simulink model "DoubleAdaptiveCBF3D"  (R2019a)
settings: Solver=ode4  StartTime=0.0  StopTime=80  FixedStep=0.001  RelTol=1e-3
values from neighbouring files (symbols this model uses):
  ddK_est0 = zeros(n,1)    [init6CBF3D.m]
  ddpref_est0 = zeros(3*n,1)    [init6CBF3D.m]
  dK0 = zeros(n,1)    [init6CBF3D.m]
  dK_est0 = zeros(n,1)    [init6CBF3D.m]
  dp0 = zeros(3*n,1)    [init6CBF3D.m]
  dpref0 = zeros(3*n,1)    [init6CBF3D.m]
  dpref_est0 = zeros(3*n,1)    [init6CBF3D.m]
  K0 = ones(n,1)    [init6CBF3D.m]
  K_est0 = ones(n,1)    [init6CBF3D.m]
  K_min = 0.3    [init6CBF3D.m]
  K_ref = 1    [init6CBF3D.m]
  obss = [ 15  16 -5  19   0  8  4 ... (first row only)    [init6CBF3D.m]
  p0 = rand(3*n,1)    [init6CBF3D.m]
  pd = reshape(pd',3*n,1)    [init6CBF3D.m]
  pref0 = zeros(3*n,1)    [init6CBF3D.m]
  pref_est0 = zeros(3*n,1)    [init6CBF3D.m]
  topology = sign(abs(LL))    [init6CBF3D.m]
libraries: commchan3 x1, cstblocks x1
settings Model: Creator=zxz  LastModifiedBy=zxz

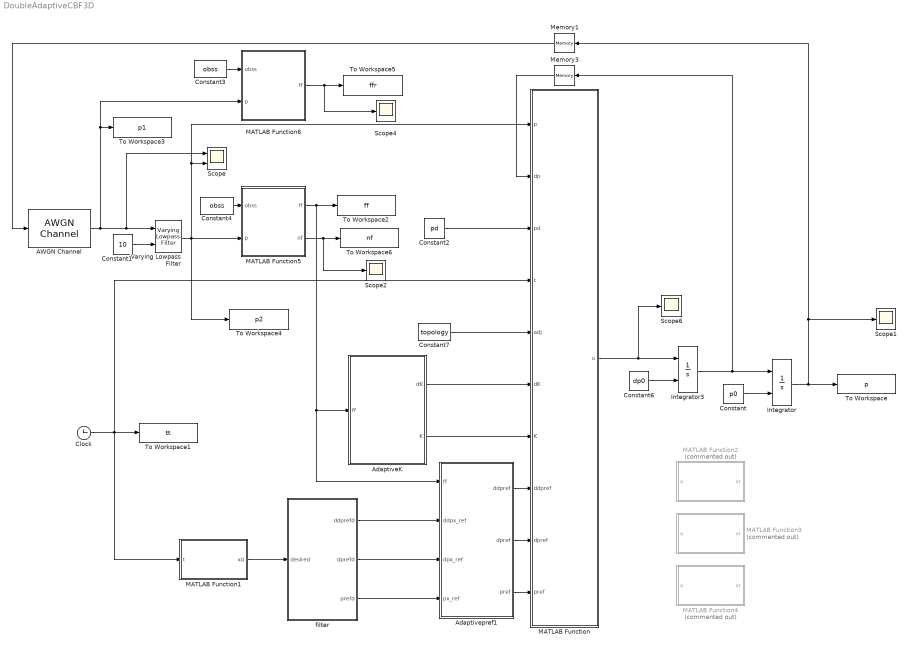
== system DoubleAdaptiveCBF3D ==
  AWGN Channel : commchan3/AWGN Channel  InputProcessing=Columns as channels (frame based)  seed=67  noiseMode="Signal to noise ratio  (Eb/No)"  EbNodB=65  EsNodB=10  SNRdB=10  bitsPerSym=1  Ps=1  Tsym=1  variance=1
      settings: SourceProductName=Communications Toolbox
  AdaptiveK : Subsystem
  Adaptivepref1 : Subsystem
  Clock : Clock
  Constant : Constant  Value=p0
  Constant1 : Constant  Value=10
  Constant2 : Constant  Value=pd
  Constant3 : Constant  Value=obss
  Constant4 : Constant  Value=obss
  Constant6 : Constant  Value=dp0
  Constant7 : Constant  Value=topology
  Integrator : Integrator  InitialConditionSource=external
  Integrator3 : Integrator  InitialConditionSource=external
  MATLAB Function : MATLAB Function  TreatAsAtomicUnit=on
  MATLAB Function1 : MATLAB Function  TreatAsAtomicUnit=on
  MATLAB Function2 : MATLAB Function  Commented=on  TreatAsAtomicUnit=on
  MATLAB Function3 : MATLAB Function  Commented=on  TreatAsAtomicUnit=on
  MATLAB Function4 : MATLAB Function  Commented=on  TreatAsAtomicUnit=on
  MATLAB Function5 : MATLAB Function  TreatAsAtomicUnit=on
  MATLAB Function6 : MATLAB Function  TreatAsAtomicUnit=on
  Memory1 : Memory
  Memory3 : Memory
  Scope : Scope  NumInputPorts=2
  Scope{1..2,4,6} (4 alike) : Scope
  To Workspace : ToWorkspace  VariableName=p  SampleTime=-1
  To Workspace1 : ToWorkspace  VariableName=tt  SampleTime=-1
  To Workspace2 : ToWorkspace  VariableName=ff  SampleTime=-1
  To Workspace3 : ToWorkspace  VariableName=p1  SampleTime=-1
  To Workspace4 : ToWorkspace  VariableName=p2  SampleTime=-1
  To Workspace5 : ToWorkspace  VariableName=ffr  SampleTime=-1
  To Workspace6 : ToWorkspace  VariableName=nf  SampleTime=-1
  Varying Lowpass Filter : cstblocks/Linear Parameter Varying/Varying Lowpass Filter  N=1
      settings: SourceProductName=Control System Toolbox
  filter : Subsystem
  wires:
  Constant/1 -> Integrator/2
  Constant2/1 -> MATLAB Function/3(pd)
  Clock/1 -> To Workspace1/1, MATLAB Function1/1(t), MATLAB Function/4(t)
  Integrator/1 -> To Workspace/1, Memory1/1, Scope1/1
  Constant7/1 -> MATLAB Function/5(adj)
  MATLAB Function1/1(xd) -> filter/1(desired)
  Memory1/1 -> AWGN Channel/1
  Constant6/1 -> Integrator3/2
  MATLAB Function/1(u) -> Scope6/1, Integrator3/1
  Integrator3/1 -> Memory3/1, Integrator/1
  Memory3/1 -> MATLAB Function/2(dp)
  Constant4/1 -> MATLAB Function5/1(obss)
  MATLAB Function5/1(ff) -> Adaptivepref1/1(ff), AdaptiveK/1(ff), To Workspace2/1
  AdaptiveK/1(dK) -> MATLAB Function/6(dK)
  AdaptiveK/2(K) -> MATLAB Function/7(K)
  Adaptivepref1/1(ddpref) -> MATLAB Function/8(ddpref)
  Adaptivepref1/2(dpref) -> MATLAB Function/9(dpref)
  Adaptivepref1/3(pref) -> MATLAB Function/10(pref)
  filter/3(prefd) -> Adaptivepref1/4(px_ref)
  filter/2(dprefd) -> Adaptivepref1/3(dpx_ref)
  filter/1(ddprefd) -> Adaptivepref1/2(ddpx_ref)
  Varying Lowpass Filter/1 -> To Workspace4/1, MATLAB Function/1(p), Scope/2, MATLAB Function5/2(p)
  Constant1/1 -> Varying Lowpass Filter/2
  AWGN Channel/1 -> MATLAB Function6/2(p), To Workspace3/1, Scope/1, Varying Lowpass Filter/1
  MATLAB Function6/1(ff) -> Scope4/1, To Workspace5/1
  Constant3/1 -> MATLAB Function6/1(obss)
  MATLAB Function5/2(nf) -> Scope2/1, To Workspace6/1

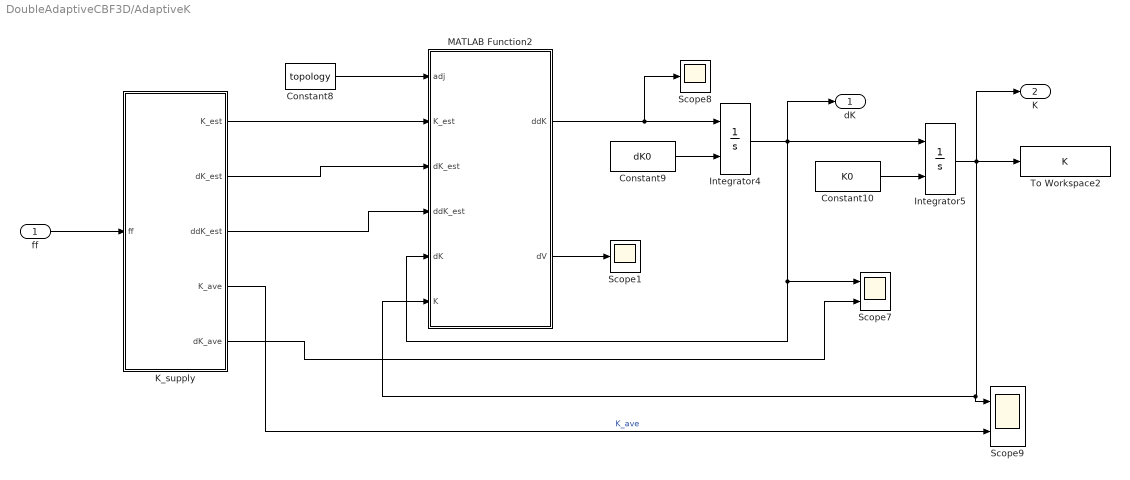
== system DoubleAdaptiveCBF3D/AdaptiveK ==
  ff : Inport
  Constant10 : Constant  Value=K0
  Constant8 : Constant  Value=topology
  Constant9 : Constant  Value=dK0
  Integrator4 : Integrator  InitialConditionSource=external
  Integrator5 : Integrator  InitialConditionSource=external
  K_supply : Subsystem
  MATLAB Function2 : MATLAB Function  TreatAsAtomicUnit=on
  Scope1 : Scope
  Scope7 : Scope  NumInputPorts=2
  Scope8 : Scope
  Scope9 : Scope  NumInputPorts=2
  To Workspace2 : ToWorkspace  VariableName=K  SampleTime=-1
  dK : Outport
  K : Outport  Port=2
  wires:
  Integrator4/1 -> MATLAB Function2/5(dK), Scope7/1, Integrator5/1, dK/1
  MATLAB Function2/1(ddK) -> Scope8/1, Integrator4/1
  Constant9/1 -> Integrator4/2
  Constant8/1 -> MATLAB Function2/1(adj)
  Integrator5/1 -> MATLAB Function2/6(K), Scope9/1, K/1, To Workspace2/1
  K_supply/1(K_est) -> MATLAB Function2/2(K_est)
  Constant10/1 -> Integrator5/2
  K_supply/3(ddK_est) -> MATLAB Function2/4(ddK_est)
  K_supply/2(dK_est) -> MATLAB Function2/3(dK_est)
  ff/1 -> K_supply/1(ff)
  K_supply/4(K_ave) -> Scope9/2  "K_ave"
  K_supply/5(dK_ave) -> Scope7/2
  MATLAB Function2/2(dV) -> Scope1/1

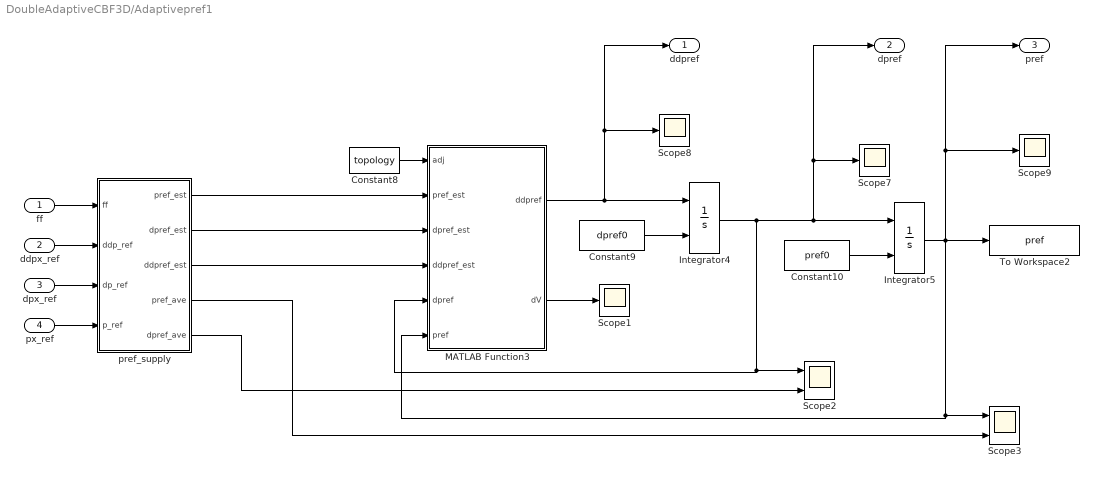
== system DoubleAdaptiveCBF3D/Adaptivepref1 ==
  ff : Inport
  ddpx_ref : Inport  Port=2
  dpx_ref : Inport  Port=3
  px_ref : Inport  Port=4
  Constant10 : Constant  Value=pref0
  Constant8 : Constant  Value=topology
  Constant9 : Constant  Value=dpref0
  Integrator4 : Integrator  InitialConditionSource=external
  Integrator5 : Integrator  InitialConditionSource=external
  MATLAB Function3 : MATLAB Function  TreatAsAtomicUnit=on
  Scope{1,7..9} (4 alike) : Scope
  Scope2 : Scope  NumInputPorts=2
  Scope3 : Scope  NumInputPorts=2
  To Workspace2 : ToWorkspace  VariableName=pref  SampleTime=-1
  pref_supply : Subsystem
  ddpref : Outport
  dpref : Outport  Port=2
  pref : Outport  Port=3
  wires:
  pref_supply/3(ddpref_est) -> MATLAB Function3/4(ddpref_est)
  Integrator4/1 -> MATLAB Function3/5(dpref), Scope2/1, dpref/1, Scope7/1, Integrator5/1
  pref_supply/2(dpref_est) -> MATLAB Function3/3(dpref_est)
  MATLAB Function3/1(ddpref) -> ddpref/1, Scope8/1, Integrator4/1
  Integrator5/1 -> Scope3/1, MATLAB Function3/6(pref), Scope9/1, pref/1, To Workspace2/1
  MATLAB Function3/2(dV) -> Scope1/1
  pref_supply/5(dpref_ave) -> Scope2/2
  pref_supply/1(pref_est) -> MATLAB Function3/2(pref_est)
  pref_supply/4(pref_ave) -> Scope3/2
  Constant10/1 -> Integrator5/2
  px_ref/1 -> pref_supply/4(p_ref)
  Constant9/1 -> Integrator4/2
  Constant8/1 -> MATLAB Function3/1(adj)
  dpx_ref/1 -> pref_supply/3(dp_ref)
  ddpx_ref/1 -> pref_supply/2(ddp_ref)
  ff/1 -> pref_supply/1(ff)

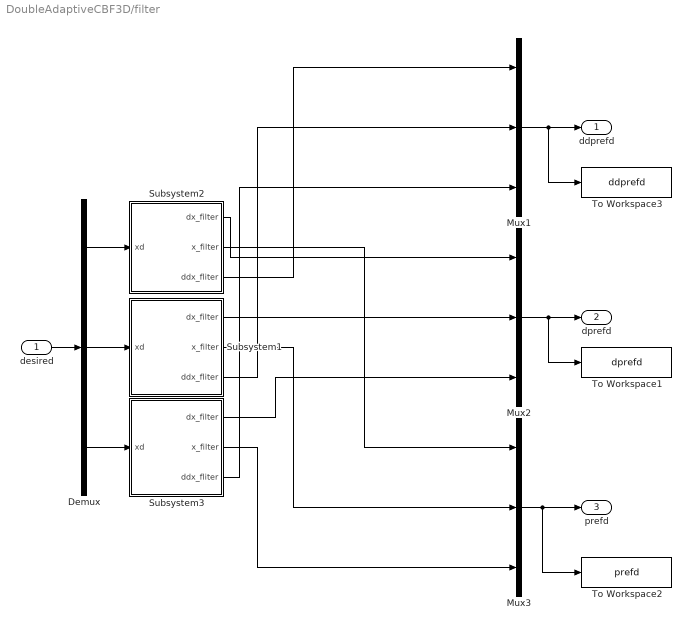
== system DoubleAdaptiveCBF3D/filter ==
  desired : Inport
  Demux : Demux  Outputs=3
  Mux1 : Mux  Inputs=3
  Mux2 : Mux  Inputs=3
  Mux3 : Mux  Inputs=3
  Subsystem1 : Subsystem
  Subsystem2 : Subsystem
  Subsystem3 : Subsystem
  To Workspace1 : ToWorkspace  VariableName=dprefd  SampleTime=-1
  To Workspace2 : ToWorkspace  VariableName=prefd  SampleTime=-1
  To Workspace3 : ToWorkspace  VariableName=ddprefd  SampleTime=-1
  ddprefd : Outport
  dprefd : Outport  Port=2
  prefd : Outport  Port=3
  wires:
  desired/1 -> Demux/1
  Demux/1 -> Subsystem2/1(xd)
  Demux/2 -> Subsystem1/1(xd)
  Mux1/1 -> To Workspace3/1, ddprefd/1
  Demux/3 -> Subsystem3/1(xd)
  Mux2/1 -> To Workspace1/1, dprefd/1
  Mux3/1 -> To Workspace2/1, prefd/1
  Subsystem2/2(x_filter) -> Mux3/1
  Subsystem1/2(x_filter) -> Mux3/2
  Subsystem3/2(x_filter) -> Mux3/3
  Subsystem2/3(ddx_fliter) -> Mux1/1
  Subsystem1/3(ddx_fliter) -> Mux1/2
  Subsystem3/3(ddx_fliter) -> Mux1/3
  Subsystem2/1(dx_filter) -> Mux2/1
  Subsystem1/1(dx_filter) -> Mux2/2
  Subsystem3/1(dx_filter) -> Mux2/3

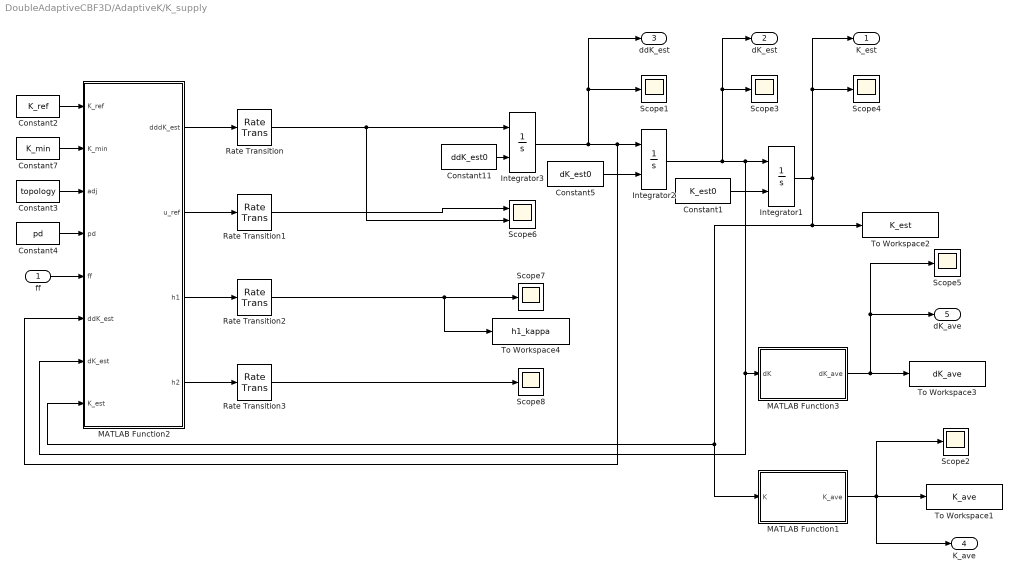
== system DoubleAdaptiveCBF3D/AdaptiveK/K_supply ==
  ff : Inport
  Constant1 : Constant  Value=K_est0
  Constant11 : Constant  Value=ddK_est0
  Constant2 : Constant  Value=K_ref
  Constant3 : Constant  Value=topology
  Constant4 : Constant  Value=pd
  Constant5 : Constant  Value=dK_est0
  Constant7 : Constant  Value=K_min
  Integrator1 : Integrator  InitialConditionSource=external
  Integrator2 : Integrator  InitialConditionSource=external
  Integrator3 : Integrator  InitialConditionSource=external
  MATLAB Function1 : MATLAB Function  TreatAsAtomicUnit=on
  MATLAB Function2 : MATLAB Function  TreatAsAtomicUnit=on
  MATLAB Function3 : MATLAB Function  TreatAsAtomicUnit=on
  Rate Transition{,1..3} (4 alike) : RateTransition
  Scope{1..5,7..8} (7 alike) : Scope
  Scope6 : Scope  NumInputPorts=2
  To Workspace1 : ToWorkspace  VariableName=K_ave  SampleTime=-1
  To Workspace2 : ToWorkspace  VariableName=K_est  SampleTime=-1
  To Workspace3 : ToWorkspace  VariableName=dK_ave  SampleTime=-1
  To Workspace4 : ToWorkspace  VariableName=h1_kappa  SampleTime=-1
  K_est : Outport
  dK_est : Outport  Port=2
  ddK_est : Outport  Port=3
  K_ave : Outport  Port=4
  dK_ave : Outport  Port=5
  wires:
  ff/1 -> MATLAB Function2/5(ff)
  Constant1/1 -> Integrator1/2
  Constant2/1 -> MATLAB Function2/1(K_ref)
  Integrator1/1 -> K_est/1, Scope4/1, To Workspace2/1, MATLAB Function1/1(K), MATLAB Function2/8(K_est)
  Constant3/1 -> MATLAB Function2/3(adj)
  Constant4/1 -> MATLAB Function2/4(pd)
  MATLAB Function1/1(K_ave) -> To Workspace1/1, K_ave/1, Scope2/1
  Constant5/1 -> Integrator2/2
  Integrator2/1 -> dK_est/1, Scope3/1, MATLAB Function2/7(dK_est), MATLAB Function3/1(dK), Integrator1/1
  MATLAB Function3/1(dK_ave) -> Scope5/1, dK_ave/1, To Workspace3/1
  Constant7/1 -> MATLAB Function2/2(K_min)
  Integrator3/1 -> Scope1/1, ddK_est/1, MATLAB Function2/6(ddK_est), Integrator2/1
  Constant11/1 -> Integrator3/2
  Rate Transition/1 -> Scope6/2, Integrator3/1
  MATLAB Function2/1(dddK_est) -> Rate Transition/1
  MATLAB Function2/2(u_ref) -> Rate Transition1/1
  Rate Transition1/1 -> Scope6/1
  MATLAB Function2/3(h1) -> Rate Transition2/1
  MATLAB Function2/4(h2) -> Rate Transition3/1
  Rate Transition3/1 -> Scope8/1
  Rate Transition2/1 -> To Workspace4/1, Scope7/1

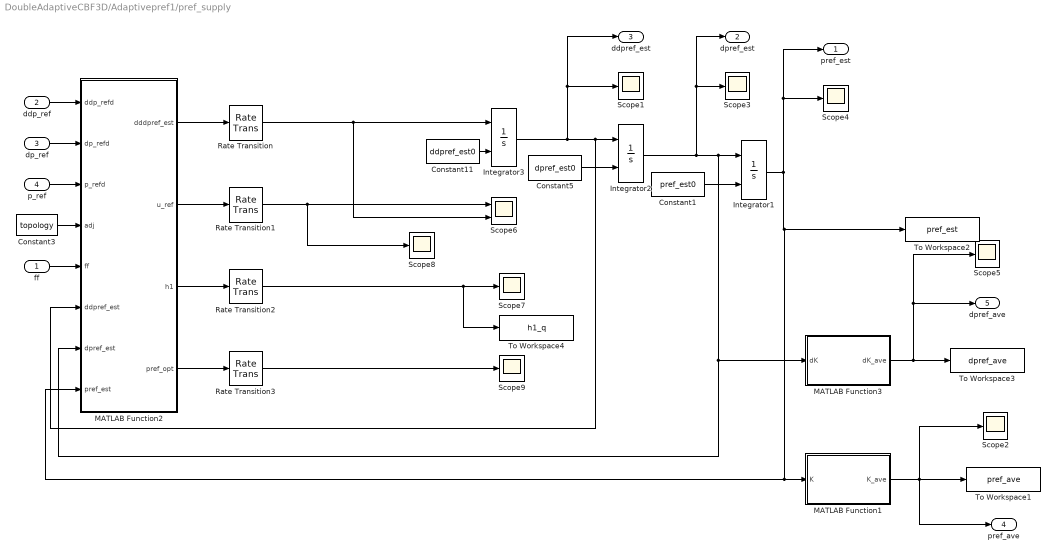
== system DoubleAdaptiveCBF3D/Adaptivepref1/pref_supply ==
  ff : Inport
  ddp_ref : Inport  Port=2
  dp_ref : Inport  Port=3
  p_ref : Inport  Port=4
  Constant1 : Constant  Value=pref_est0
  Constant11 : Constant  Value=ddpref_est0
  Constant3 : Constant  Value=topology
  Constant5 : Constant  Value=dpref_est0
  Integrator1 : Integrator  InitialConditionSource=external
  Integrator2 : Integrator  InitialConditionSource=external
  Integrator3 : Integrator  InitialConditionSource=external
  MATLAB Function1 : MATLAB Function  TreatAsAtomicUnit=on
  MATLAB Function2 : MATLAB Function  TreatAsAtomicUnit=on
  MATLAB Function3 : MATLAB Function  TreatAsAtomicUnit=on
  Rate Transition{,1..3} (4 alike) : RateTransition
  Scope{1..5,7..9} (8 alike) : Scope
  Scope6 : Scope  NumInputPorts=2
  To Workspace1 : ToWorkspace  VariableName=pref_ave  SampleTime=-1
  To Workspace2 : ToWorkspace  VariableName=pref_est  SampleTime=-1
  To Workspace3 : ToWorkspace  VariableName=dpref_ave  SampleTime=-1
  To Workspace4 : ToWorkspace  VariableName=h1_q  SampleTime=-1
  pref_est : Outport
  dpref_est : Outport  Port=2
  ddpref_est : Outport  Port=3
  pref_ave : Outport  Port=4
  dpref_ave : Outport  Port=5
  wires:
  Constant11/1 -> Integrator3/2
  Rate Transition2/1 -> To Workspace4/1, Scope7/1
  Rate Transition/1 -> Integrator3/1, Scope6/2
  MATLAB Function2/2(u_ref) -> Rate Transition1/1
  Integrator2/1 -> dpref_est/1, Scope3/1, MATLAB Function2/7(dpref_est), MATLAB Function3/1(dK), Integrator1/1
  Integrator3/1 -> Scope1/1, ddpref_est/1, MATLAB Function2/6(ddpref_est), Integrator2/1
  Constant5/1 -> Integrator2/2
  Rate Transition1/1 -> Scope8/1, Scope6/1
  Constant1/1 -> Integrator1/2
  Constant3/1 -> MATLAB Function2/4(adj)
  MATLAB Function2/3(h1) -> Rate Transition2/1
  Integrator1/1 -> To Workspace2/1, MATLAB Function1/1(K), MATLAB Function2/8(pref_est), pref_est/1, Scope4/1
  MATLAB Function1/1(K_ave) -> To Workspace1/1, pref_ave/1, Scope2/1
  MATLAB Function3/1(dK_ave) -> Scope5/1, dpref_ave/1, To Workspace3/1
  ff/1 -> MATLAB Function2/5(ff)
  MATLAB Function2/1(dddpref_est) -> Rate Transition/1
  ddp_ref/1 -> MATLAB Function2/1(ddp_refd)
  dp_ref/1 -> MATLAB Function2/2(dp_refd)
  p_ref/1 -> MATLAB Function2/3(p_refd)
  Rate Transition3/1 -> Scope9/1
  MATLAB Function2/4(pref_opt) -> Rate Transition3/1

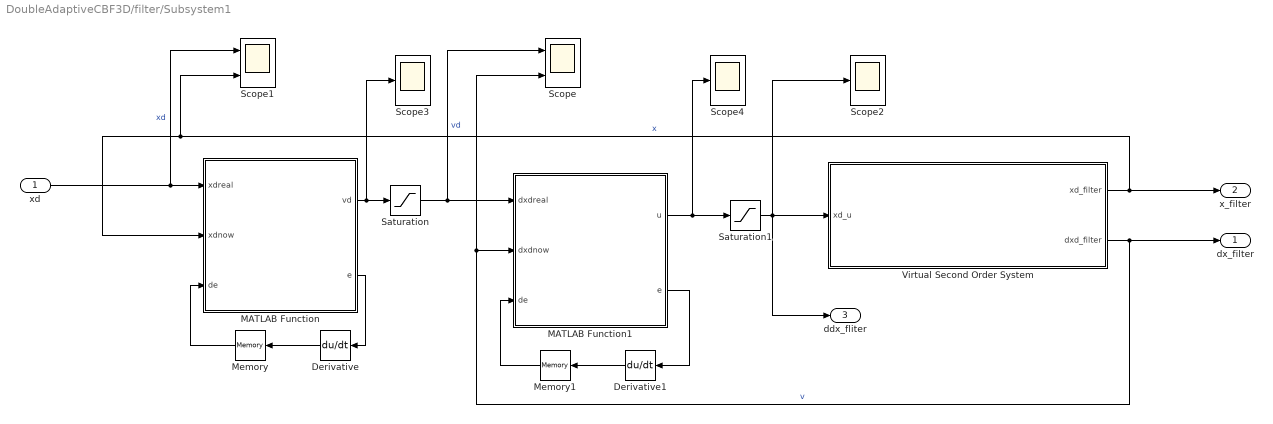
== system DoubleAdaptiveCBF3D/filter/Subsystem1 ==
  xd : Inport
  Derivative : Derivative
  Derivative1 : Derivative
  MATLAB Function : MATLAB Function  TreatAsAtomicUnit=on
  MATLAB Function1 : MATLAB Function  TreatAsAtomicUnit=on
  Memory : Memory
  Memory1 : Memory
  Saturation : Saturate  UpperLimit=2  LowerLimit=-2
  Saturation1 : Saturate  UpperLimit=1  LowerLimit=-1
  Scope : Scope  NumInputPorts=2
  Scope1 : Scope  NumInputPorts=2
  Scope2 : Scope
  Scope3 : Scope
  Scope4 : Scope
  Virtual Second Order System : Subsystem
  dx_filter : Outport
  x_filter : Outport  Port=2
  ddx_fliter : Outport  Port=3
  wires:
  MATLAB Function1/1(u) -> Scope4/1, Saturation1/1
  Saturation1/1 -> ddx_fliter/1, Scope2/1, Virtual Second Order System/1(xd_u)
  Virtual Second Order System/2(dxd_filter) -> dx_filter/1, Scope/2, MATLAB Function1/2(dxdnow)  "v"
  MATLAB Function/1(vd) -> Scope3/1, Saturation/1
  Derivative1/1 -> Memory1/1
  xd/1 -> Scope1/1, MATLAB Function/1(xdreal)  "xd"
  Saturation/1 -> Scope/1, MATLAB Function1/1(dxdreal)  "vd"
  MATLAB Function/2(e) -> Derivative/1
  Memory1/1 -> MATLAB Function1/3(de)
  Derivative/1 -> Memory/1
  Virtual Second Order System/1(xd_filter) -> MATLAB Function/2(xdnow), Scope1/2, x_filter/1  "x"
  MATLAB Function1/2(e) -> Derivative1/1
  Memory/1 -> MATLAB Function/3(de)

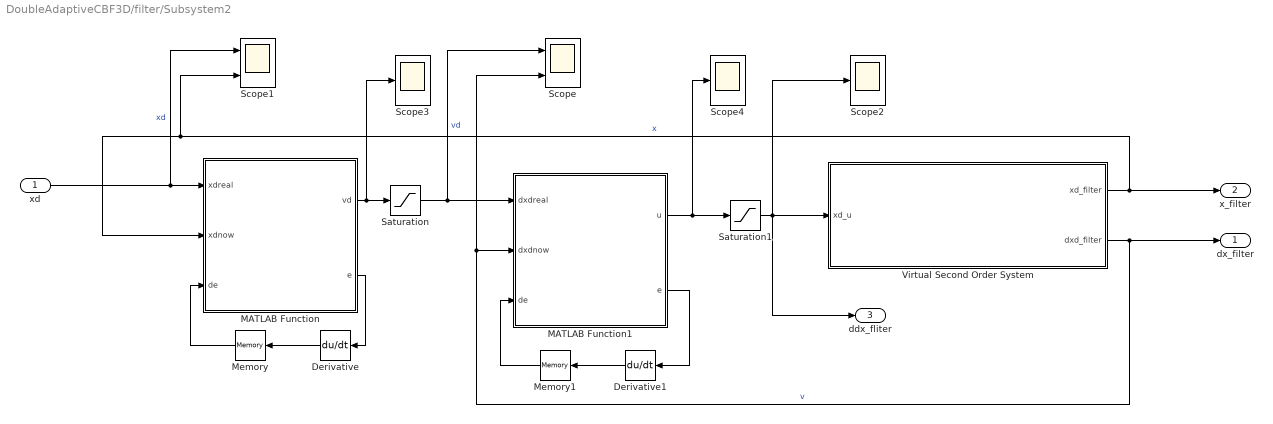
== system DoubleAdaptiveCBF3D/filter/Subsystem2 ==
  xd : Inport
  Derivative : Derivative
  Derivative1 : Derivative
  MATLAB Function : MATLAB Function  TreatAsAtomicUnit=on
  MATLAB Function1 : MATLAB Function  TreatAsAtomicUnit=on
  Memory : Memory
  Memory1 : Memory
  Saturation : Saturate  UpperLimit=1.5  LowerLimit=-1.5
  Saturation1 : Saturate  UpperLimit=1  LowerLimit=-1
  Scope : Scope  NumInputPorts=2
  Scope1 : Scope  NumInputPorts=2
  Scope2 : Scope
  Scope3 : Scope
  Scope4 : Scope
  Virtual Second Order System : Subsystem
  dx_filter : Outport
  x_filter : Outport  Port=2
  ddx_fliter : Outport  Port=3
  wires:
  MATLAB Function1/1(u) -> Scope4/1, Saturation1/1
  Saturation1/1 -> ddx_fliter/1, Scope2/1, Virtual Second Order System/1(xd_u)
  Virtual Second Order System/2(dxd_filter) -> dx_filter/1, Scope/2, MATLAB Function1/2(dxdnow)  "v"
  MATLAB Function/1(vd) -> Scope3/1, Saturation/1
  Derivative1/1 -> Memory1/1
  xd/1 -> Scope1/1, MATLAB Function/1(xdreal)  "xd"
  Saturation/1 -> Scope/1, MATLAB Function1/1(dxdreal)  "vd"
  MATLAB Function/2(e) -> Derivative/1
  Memory1/1 -> MATLAB Function1/3(de)
  Derivative/1 -> Memory/1
  Virtual Second Order System/1(xd_filter) -> MATLAB Function/2(xdnow), Scope1/2, x_filter/1  "x"
  MATLAB Function1/2(e) -> Derivative1/1
  Memory/1 -> MATLAB Function/3(de)

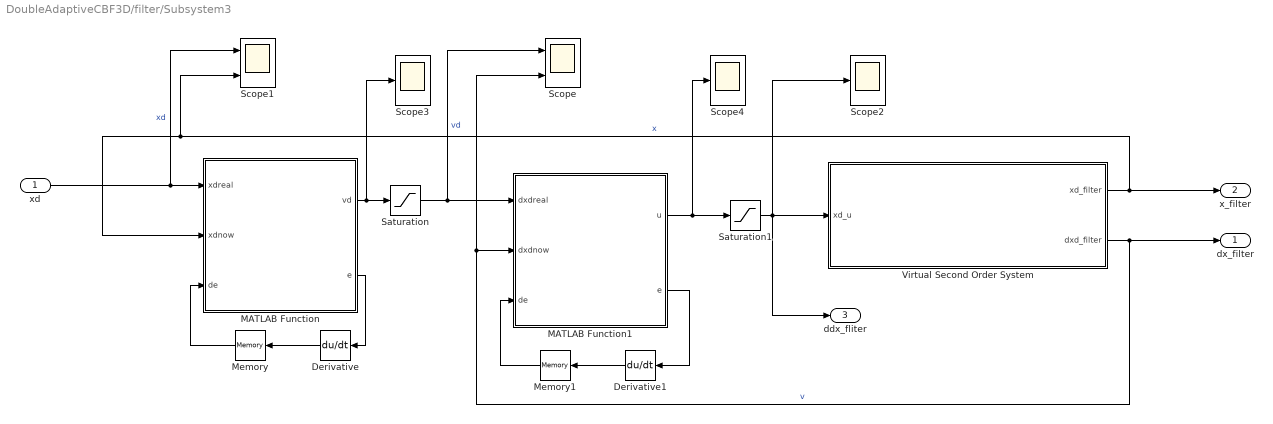
== system DoubleAdaptiveCBF3D/filter/Subsystem3 ==
  xd : Inport
  Derivative : Derivative
  Derivative1 : Derivative
  MATLAB Function : MATLAB Function  TreatAsAtomicUnit=on
  MATLAB Function1 : MATLAB Function  TreatAsAtomicUnit=on
  Memory : Memory
  Memory1 : Memory
  Saturation : Saturate  UpperLimit=2  LowerLimit=-2
  Saturation1 : Saturate  UpperLimit=1  LowerLimit=-1
  Scope : Scope  NumInputPorts=2
  Scope1 : Scope  NumInputPorts=2
  Scope2 : Scope
  Scope3 : Scope
  Scope4 : Scope
  Virtual Second Order System : Subsystem
  dx_filter : Outport
  x_filter : Outport  Port=2
  ddx_fliter : Outport  Port=3
  wires:
  MATLAB Function1/1(u) -> Scope4/1, Saturation1/1
  Saturation1/1 -> ddx_fliter/1, Scope2/1, Virtual Second Order System/1(xd_u)
  Virtual Second Order System/2(dxd_filter) -> dx_filter/1, Scope/2, MATLAB Function1/2(dxdnow)  "v"
  MATLAB Function/1(vd) -> Scope3/1, Saturation/1
  Derivative1/1 -> Memory1/1
  xd/1 -> Scope1/1, MATLAB Function/1(xdreal)  "xd"
  Saturation/1 -> Scope/1, MATLAB Function1/1(dxdreal)  "vd"
  MATLAB Function/2(e) -> Derivative/1
  Memory1/1 -> MATLAB Function1/3(de)
  Derivative/1 -> Memory/1
  Virtual Second Order System/1(xd_filter) -> MATLAB Function/2(xdnow), Scope1/2, x_filter/1  "x"
  MATLAB Function1/2(e) -> Derivative1/1
  Memory/1 -> MATLAB Function/3(de)

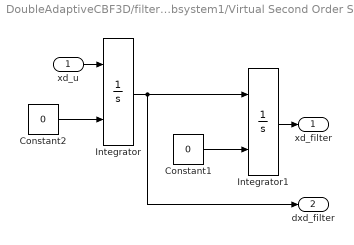
== system DoubleAdaptiveCBF3D/filter/Subsystem1/Virtual Second Order System ==
  xd_u : Inport
  Constant1 : Constant  Value=0
  Constant2 : Constant  Value=0
  Integrator : Integrator  InitialConditionSource=external
  Integrator1 : Integrator  InitialConditionSource=external
  xd_filter : Outport  VectorParamsAs1DForOutWhenUnconnected=on
  dxd_filter : Outport  Port=2  VectorParamsAs1DForOutWhenUnconnected=on
  wires:
  Constant1/1 -> Integrator1/2
  Integrator/1 -> dxd_filter/1, Integrator1/1
  Constant2/1 -> Integrator/2
  xd_u/1 -> Integrator/1
  Integrator1/1 -> xd_filter/1

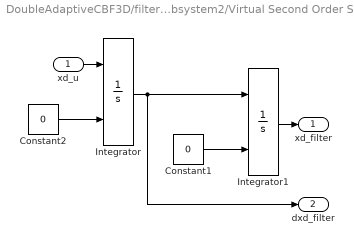
== system DoubleAdaptiveCBF3D/filter/Subsystem2/Virtual Second Order System ==
  xd_u : Inport
  Constant1 : Constant  Value=0
  Constant2 : Constant  Value=0
  Integrator : Integrator  InitialConditionSource=external
  Integrator1 : Integrator  InitialConditionSource=external
  xd_filter : Outport  VectorParamsAs1DForOutWhenUnconnected=on
  dxd_filter : Outport  Port=2  VectorParamsAs1DForOutWhenUnconnected=on
  wires:
  Constant1/1 -> Integrator1/2
  Integrator/1 -> dxd_filter/1, Integrator1/1
  Constant2/1 -> Integrator/2
  xd_u/1 -> Integrator/1
  Integrator1/1 -> xd_filter/1

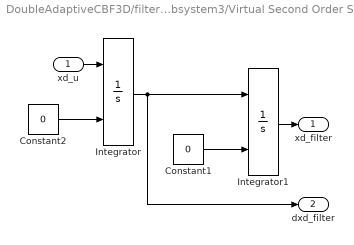
== system DoubleAdaptiveCBF3D/filter/Subsystem3/Virtual Second Order System ==
  xd_u : Inport
  Constant1 : Constant  Value=0
  Constant2 : Constant  Value=0
  Integrator : Integrator  InitialConditionSource=external
  Integrator1 : Integrator  InitialConditionSource=external
  xd_filter : Outport  VectorParamsAs1DForOutWhenUnconnected=on
  dxd_filter : Outport  Port=2  VectorParamsAs1DForOutWhenUnconnected=on
  wires:
  Constant1/1 -> Integrator1/2
  Integrator/1 -> dxd_filter/1, Integrator1/1
  Constant2/1 -> Integrator/2
  xd_u/1 -> Integrator/1
  Integrator1/1 -> xd_filter/1

== matlab function DoubleAdaptiveCBF3D/filter/Subsystem2/MATLAB Function ==
  data: xdreal input; vd output; xdnow input; de input; e output
function [vd,e] = Position_Control(xdreal,xdnow,de)
kp = 1;
kd = 0.1;

e=xdreal-xdnow;

vd = kp*e+kd*de;

== matlab function DoubleAdaptiveCBF3D/MATLAB Function ==
  data: p input; dp input; u output; pd input; t input; adj input; dK input; K input; ddpref input; dpref input; pref input
function u   = control(p,dp,pd,t,adj,dK,K,ddpref,dpref,pref)

u  = zeros(length(p),1);

%% formation 
k0=3;
k1=3;
for i=1:length(p)/3
    u((i-1)*3+1:(i-1)*3+3) = u((i-1)*3+1:(i-1)*3+3) + ddpref((i-1)*3+1:(i-1)*3+3);
    u((i-1)*3+1:(i-1)*3+3) = u((i-1)*3+1:(i-1)*3+3) - k1*(p((i-1)*3+1:(i-1)*3+3)-(pref((i-1)*3+1:(i-1)*3+3)+K(i)*pd((i-1)*3+1:(i-1)*3+3)));
    u((i-1)*3+1:(i-1)*3+3) = u((i-1)*3+1:(i-1)*3+3) - k1*(dp((i-1)*3+1:(i-1)*3+3)-(dpref((i-1)*3+1:(i-1)*3+3)+dK(i)*pd((i-1)*3+1:(i-1)*3+3)));
    for j=1:length(p)/3
        if(i==j) continue;
        end
        rij  = p((i-1)*3+1:(i-1)*3+3)-p((j-1)*3+1:(j-1)*3+3);
        drij = dp((i-1)*3+1:(i-1)*3+3)-dp((j-1)*3+1:(j-1)*3+3);
        rijd = pd((i-1)*3+1:(i-1)*3+3)-pd((j-1)*3+1:(j-1)*3+3);
        u((i-1)*3+1:(i-1)*3+3) = u((i-1)*3+1:(i-1)*3+3) - k0*adj(i,j)*(rij+drij);
        u((i-1)*3+1:(i-1)*3+3) = u((i-1)*3+1:(i-1)*3+3) - k1*adj(i,j)*((rij-K(i)*rijd)+(drij-dK(i)*rijd));
    end
end


end

== matlab function DoubleAdaptiveCBF3D/filter/Subsystem1/MATLAB Function ==
  data: xdreal input; vd output; xdnow input; de input; e output
function [vd,e] = Position_Control(xdreal,xdnow,de)
kp = 1;
kd = 0.1;

e=xdreal-xdnow;

vd = kp*e+kd*de;

== matlab function DoubleAdaptiveCBF3D/MATLAB Function1 ==
  data: t input; xd output
function xd  = Desired_Position(t)
xd=[0 0 0]';

if(t>15)
    xd=[70 0 0]';
end


end

== matlab function DoubleAdaptiveCBF3D/AdaptiveK/K_supply/MATLAB Function2 ==
  settings: updateMethod=DISCRETE  sampleTime=0.01
  data: dddK_est output; K_ref input; K_min input; adj input; pd input; ff input; ddK_est input; dK_est input; K_est input; u_ref output; h1 output; h2 output
function [dddK_est,u_ref,h1,h2]  = K_supply(K_ref,K_min,adj,pd,ff,ddK_est,dK_est,K_est)

dddK_est  = zeros(length(ff)/3,1);
u_ref     = zeros(length(ff)/3,1);
h1        = zeros(length(ff)/3,1);
h2        = zeros(length(ff)/3,1);

miu=1.5;

a=2.8363;b=2.0111;

delta1=1.5;delta2=1.4087;delta3=1.4276;

gamma=1;
k1=10;
kk=70;

A=zeros(2,2);
B=zeros(2,1);
Aeq=zeros(1,2);
Beq=zeros(1,1);
H=[1 -1,
  -1 1];


coder.extrinsic('QPref');
for i=1:length(ff)/3
    
    K_opt=ff(3*(i-1)+1:3*(i-1)+3)'*pd((i-1)*2+1:(i-1)*2+3)/norm(pd((i-1)*2+1:(i-1)*2+3));
    
    h1(i) = miu^2-(ddK_est(i)+a*dK_est(i)+b*(K_est(i)-K_min)).^2;
    h2(i) = K_est(i)-K_min;
    
    s        = ddK_est(i)+a*dK_est(i)+b*(K_est(i)-K_ref);
    
    if(K_opt>=0)
        dddK_est(i)=-k1*s-a*ddK_est(i)-b*dK_est(i);
        continue;
    end
    
    u_ref(i) = -k1*s-a*ddK_est(i)-b*dK_est(i)+kk*K_opt;
%     u_ref(i) = -k1*s-a*ddK_est(i)-b*dK_est(i);
    
    A  = [2*(ddK_est(i)+a*dK_est(i)+b*(K_est(i)-K_min)) 0, 
                                                    -1  0];
           
    B(1) = -2*(ddK_est(i)+a*dK_est(i)+b*(K_est(i)-K_min))*(a*ddK_est(i)+b*dK_est(i)) ...
         +gamma*(miu^2-(ddK_est(i)+a*dK_est(i)+b*(K_est(i)-K_min))^2);
    B(2) = (delta1+delta2+delta3)*ddK_est(i) ...
         +(delta2*delta1+delta3*delta1+delta3*delta2)*dK_est(i) ...
         +delta1*delta2*delta3*(K_est(i)-K_min);
    
    Aeq    = [0 1];
    Beq(1) = u_ref(i);
    x_ans = zeros(2,1);
    exitflag = zeros(1);
    [x_ans,~,exitflag] = QPref(A,[0 0]',B,H,Aeq,Beq);
%     [x_ans,~,exitflag] = quadprog(H,[0 0]',A,B,Aeq,beq,ws);
    if(exitflag==-2)
        char('zxzerror')
    end
    
%     dddK_est(i) = u_ref(i);
    dddK_est(i) = x_ans(1);
    
end


end

== matlab function DoubleAdaptiveCBF3D/AdaptiveK/K_supply/MATLAB Function1 ==
  data: K input; K_ave output
function K_ave  = Kaver(K)

K_ave=sum(K)/length(K);

end

== matlab function DoubleAdaptiveCBF3D/MATLAB Function2 ==
  data: x input; xr output
function xr  = Desired_Position(x)
n=7;
xr=zeros(3*n,1);
for i=1:n
    xr(3*(i-1)+1:3*(i-1)+3)=x;
end

end

== matlab function DoubleAdaptiveCBF3D/MATLAB Function3 ==
  data: x input; xr output
function xr  = Desired_Position(x)
n=7;
xr=zeros(3*n,1);
for i=1:n
    xr(3*(i-1)+1:3*(i-1)+3)=x;
end

end

== matlab function DoubleAdaptiveCBF3D/filter/Subsystem2/MATLAB Function1 ==
  data: dxdreal input; u output; dxdnow input; de input; e output
function [u,e] = Velocity_Control(dxdreal,dxdnow,de)
kp = 5;
kd = 0.1;

e=dxdreal-dxdnow;

u = kp*e+kd*de;

== matlab function DoubleAdaptiveCBF3D/filter/Subsystem1/MATLAB Function1 ==
  data: dxdreal input; u output; dxdnow input; de input; e output
function [u,e] = Velocity_Control(dxdreal,dxdnow,de)
kp = 5;
kd = 0.1;

e=dxdreal-dxdnow;

u = kp*e+kd*de;

== matlab function DoubleAdaptiveCBF3D/AdaptiveK/MATLAB Function2 ==
  data: adj input; K_est input; dK_est input; ddK_est input; ddK output; dK input; K input; dV output
function [ddK, dV]   = GetK(adj,K_est,dK_est,ddK_est,dK,K)
ddK = zeros(length(K_est),1);

k3=2;
beta=1;
fai=10;
a=2.8363;b=2.0111;
dV=0;

for i=1:length(K_est)
    ddK(i) = ddK(i) + ddK_est(i) - a*(dK(i)-dK_est(i)) -b*(K(i)-K_est(i));
    s1=0;
    s2=0;
    for j=1:length(K_est)
        if(i==j||adj(i,j)<0.5) continue;
        end
        sg1=K(i)-K(j);
        sg2=dK(i)-dK(j);
%         ddK(i) = ddK(i) - fai*mysign(sg1)-fai*sg2;
%         ddK(i) = ddK(i) - fai*mysign(sg1)*abs(sg1)^1.2-fai*sg2;
%         ddK(i) = ddK(i) - 10*sg1-fai*sign(sg2);
%         ddK(i) = ddK(i) -beta*fai*mysign(sg1+sg2);
%         ddK(i) = ddK(i) -40*sign(sg1)-fai*sign(sg2);
        ddK(i) = ddK(i) -200*sign(sg1)-100*sign(sg2);
%         dV=dV+sg2^2;
    end
%     ddK(i) = ddK(i) - fai*sign(s1)-fai*sign(s2);

end
% ddK = zeros(length(K_est),1);
end

== matlab function DoubleAdaptiveCBF3D/MATLAB Function6 ==
  data: obss input; ff output; p input
function ff  = Desired_Position(obss,p)

kf=1;


ff=zeros(length(p),1);
for i=1:length(p)/3
    dis=5;
    fmain=[0 0 0]';
    ff(3*(i-1)+1:3*(i-1)+3)=fmain;
    for j=1:length(obss(:,1))
        a = obss(j,4:6)-obss(j,1:3);
        b = p(3*(i-1)+1:3*(i-1)+3,1)'-obss(j,1:3);
            
        proj = a*b'./norm(a);
        ftmp    = (b-proj*a./norm(a));
        disf    = norm(ftmp)-obss(j,7);
        if(disf<dis)
            dis=disf;
            fmain=ftmp;
            ff(3*(i-1)+1:3*(i-1)+3)=kf*fmain./norm(fmain);
        end
    end
end

end

== matlab function DoubleAdaptiveCBF3D/AdaptiveK/K_supply/MATLAB Function3 ==
  data: dK input; dK_ave output
function dK_ave  = dKaver(dK)

dK_ave=sum(dK)/length(dK);

end

== matlab function DoubleAdaptiveCBF3D/MATLAB Function4 ==
  data: x input; xr output
function xr  = Desired_Position(x)
n=7;
xr=zeros(3*n,1);
for i=1:n
    xr(3*(i-1)+1:3*(i-1)+3)=x;
end

end

== matlab function DoubleAdaptiveCBF3D/MATLAB Function5 ==
  data: obss input; ff output; p input; nf output
function [ff,nf]  = Desired_Position(obss,p)

kf=1;


ff=zeros(length(p),1);
nf=zeros(length(p)/3,1);
for i=1:length(p)/3
    dis=5;
    fmain=[0 0 0]';
    ff(3*(i-1)+1:3*(i-1)+3)=fmain;
    for j=1:length(obss(:,1))
        a = obss(j,4:6)-obss(j,1:3);
        b = p(3*(i-1)+1:3*(i-1)+3,1)'-obss(j,1:3);
            
        proj = a*b'./norm(a);
        ftmp    = (b-proj*a./norm(a));
        disf    = norm(ftmp)-obss(j,7);
        if(disf<dis)
            dis=disf;
            fmain=ftmp;
            ff(3*(i-1)+1:3*(i-1)+3)=kf*fmain./norm(fmain);
        end
    end
    nf(i)=norm(ff(3*(i-1)+1:3*(i-1)+3));
end

end

== matlab function DoubleAdaptiveCBF3D/Adaptivepref1/MATLAB Function3 ==
  data: adj input; pref_est input; dpref_est input; ddpref output; ddpref_est input; dpref input; pref input; dV output
function [ddpref, dV]   = GetK(adj,pref_est,dpref_est,ddpref_est,dpref,pref)
ddpref = zeros(length(pref_est),1);

k3=2;
beta=1;
fai=20;
a=2.8363;b=2.0111;
dV=0;

for i=1:length(pref_est)/3
    ddpref(3*(i-1)+1:3*(i-1)+3) =  ddpref_est(3*(i-1)+1:3*(i-1)+3) ... 
        -a*(dpref(3*(i-1)+1:3*(i-1)+3)-dpref_est(3*(i-1)+1:3*(i-1)+3)) ...
        -b*(pref(3*(i-1)+1:3*(i-1)+3)-pref_est(3*(i-1)+1:3*(i-1)+3));
    s1=0;
    s2=0;
    for j=1:length(pref_est)/3
        if(i==j||adj(i,j)<0.5) continue;
        end
        sg1 = pref(3*(i-1)+1:3*(i-1)+3)  - pref(3*(j-1)+1:3*(j-1)+3);
        sg2 = dpref(3*(i-1)+1:3*(i-1)+3) - dpref(3*(j-1)+1:3*(j-1)+3);
%         ddK(i) = ddK(i) - fai*mysign(sg1)-fai*sg2;
%         ddK(i) = ddK(i) - fai*mysign(sg1)*abs(sg1)^1.2-fai*sg2;
%         ddK(i) = ddK(i) - 10*sg1-fai*sign(sg2);
%         ddK(i) = ddK(i) -beta*fai*mysign(sg1+sg2);
%         ddpref(3*(i-1)+1:3*(i-1)+3) = ddpref(3*(i-1)+1:3*(i-1)+3) -20*sign(sg1)-fai*sign(sg2);
        ddpref(3*(i-1)+1:3*(i-1)+3) = ddpref(3*(i-1)+1:3*(i-1)+3) -600*sign(sg1)-300*sign(sg2);
%         dV=dV+sg2^2;
    end
%     ddK(i) = ddK(i) - fai*sign(s1)-fai*sign(s2);

end
% ddK = zeros(length(K_est),1);
end

== matlab function DoubleAdaptiveCBF3D/Adaptivepref1/pref_supply/MATLAB Function1 ==
  data: K input; K_ave output
function K_ave  = Kaver(K)

sumer=[0 0 0]';
for i=1:length(K)/3
    sumer=sumer+K(3*(i-1)+1:3*(i-1)+3);
end
K_ave=sumer./(length(K)/3);

end

== matlab function DoubleAdaptiveCBF3D/Adaptivepref1/pref_supply/MATLAB Function2 ==
  settings: updateMethod=DISCRETE  sampleTime=0.01
  data: dddpref_est output; ddp_refd input; dp_refd input; p_refd input; adj input; ff input; ddpref_est input; dpref_est input; pref_est input; u_ref output; h1 output; pref_opt output
function [dddpref_est,u_ref,h1,pref_opt]  = K_supply(ddp_refd,dp_refd,p_refd,adj,ff,ddpref_est,dpref_est,pref_est)

dddpref_est  = zeros(length(ff),1);
u_ref         = zeros(length(ff),1);
h1            = zeros(length(ff)/3,1);

miu=7;

a=2.8363;b=2.0111;

gamma=1;
k1=10;
kk=70;
A=zeros(1,3);
B=zeros(1,1);
Aeq=zeros(6,6);
Beq=zeros(3,1);
H1=[1 -1,
  -1 1];
H=kron(H1,diag([1 1 1]));


coder.extrinsic('QPref');

for i=1:length(ff)/3
    pref_opt = ff(3*(i-1)+1:3*(i-1)+3);
    ddq = ddpref_est(3*(i-1)+1:3*(i-1)+3);
    dq  = dpref_est(3*(i-1)+1:3*(i-1)+3);
    q   = pref_est(3*(i-1)+1:3*(i-1)+3);
    
    
%     s     = (ddq-ddp_refd)+a*(dq-dp_refd)+b*(q-p_refd);
    s     = (ddq)+a*(dq-dp_refd)+b*(q-p_refd);
    h1(i) = miu^2-norm(s)^2;
%     u_ref(3*(i-1)+1:3*(i-1)+3) = -k1*s-a*(ddq-ddp_refd)-b*(dq-dp_refd)+kk*pref_opt;
    u_ref(3*(i-1)+1:3*(i-1)+3) = -k1*s-a*(ddq-ddp_refd)-b*(dq-dp_refd)+kk*pref_opt;

    if(norm(ff(3*(i-1)+1:3*(i-1)+3))<=0.1)
%         dddpref_est(3*(i-1)+1:3*(i-1)+3) = -k1*s+ddp_refd-a*(ddq-ddp_refd)-b*(dq-dp_refd);
        dddpref_est(3*(i-1)+1:3*(i-1)+3) = -k1*s-a*(ddq-ddp_refd)-b*(dq-dp_refd);
        continue;
    end
    
    A  = [2*s' 0 0 0];
           
    B = -2*s'*(a*(ddq-ddp_refd)+b*(dq-dp_refd)) ...
         +gamma*h1(i);
    
    Aeq  = kron([0 1],diag([1 1 1]));
    Beq = u_ref(3*(i-1)+1:3*(i-1)+3);
    x_ans = zeros(6,1);
    exitflag = zeros(1);
    [x_ans,~,exitflag] = QPref(A,zeros(1,6),B,H,Aeq,Beq);
    if(exitflag==-2)
        char('zxzerror')
    end
    
%     dddpxref_est(i) = u_ref(i);
    dddpref_est(3*(i-1)+1:3*(i-1)+3) = x_ans(1:3);
    
end


end

== matlab function DoubleAdaptiveCBF3D/filter/Subsystem3/MATLAB Function ==
  data: xdreal input; vd output; xdnow input; de input; e output
function [vd,e] = Position_Control(xdreal,xdnow,de)
kp = 1;
kd = 0.1;

e=xdreal-xdnow;

vd = kp*e+kd*de;

== matlab function DoubleAdaptiveCBF3D/filter/Subsystem3/MATLAB Function1 ==
  data: dxdreal input; u output; dxdnow input; de input; e output
function [u,e] = Velocity_Control(dxdreal,dxdnow,de)
kp = 5;
kd = 0.1;

e=dxdreal-dxdnow;

u = kp*e+kd*de;

== matlab function DoubleAdaptiveCBF3D/Adaptivepref1/pref_supply/MATLAB Function3 ==
  data: dK input; dK_ave output
function dK_ave  = dKaver(dK)

sumer=[0 0 0]';
for i=1:length(dK)/3
    sumer=sumer+dK(3*(i-1)+1:3*(i-1)+3);
end
dK_ave=sumer./(length(dK)/3);

end
